simulink model "car_control"  (R2022b)
settings: Solver=VariableStepAuto  StartTime=0.0  StopTime=30  RelTol=1e-3
undefined symbols (not defined in the file): m, r
settings Model: Creator=The MathWorks, Inc.  LastModifiedBy=wzy19
settings SolverCC: AlgebraicLoopSolver=TrustRegion
settings DataIOCC: ReturnWorkspaceOutputs=off
settings DebuggingCC: BusObjectLabelMismatch=none  RootOutportRequireBusObject=none  PregeneratedLibrarySubsystemCodeDiagnostic=none  SFMachineParentedDataDiag=warning  ArithmeticOperatorsInVariantConditions=warning
settings ModelReferenceCC: EnableRefExpFcnMdlSchedulingChecks=on
settings SFSimCC: SimUseLocalCustomCode=off
settings RTWCC: RTWUseLocalCustomCode=off

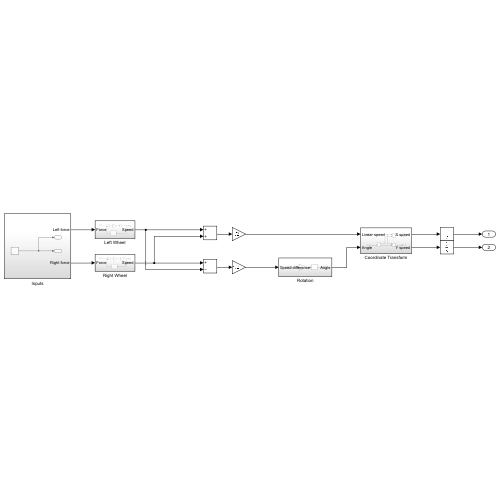
[thumbnail: Simulink's stored preview of the top-level diagram]
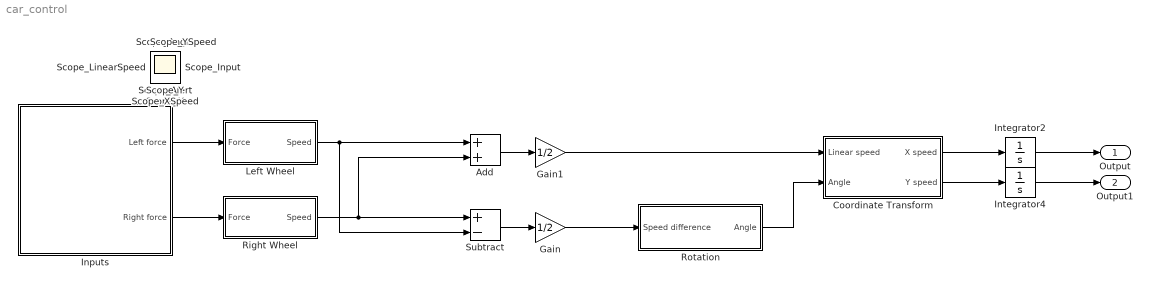
== system car_control ==
  Add : Sum
  Coordinate Transform : Subsystem
  Gain : Gain  Gain=1/2
  Gain1 : Gain  Gain=1/2
  Inputs : Subsystem
  Integrator2 : Integrator
  Integrator4 : Integrator
  Left Wheel : Subsystem
  Right Wheel : Subsystem
  Rotation : Subsystem
  Subtract : Sum  Inputs=+-
  Output : Outport
  Output1 : Outport  Port=2
  Scope_Alert : Scope
  Scope_Angle : Scope
  Scope_Input : Scope
  Scope_LinearSpeed : Scope
  Scope_X : Scope
  Scope_XSpeed : Scope
  Scope_Y : Scope
  Scope_YSpeed : Scope
  wires:
  Coordinate Transform/1(X speed) -> Integrator2/1
  Coordinate Transform/2(Y speed) -> Integrator4/1
  Left Wheel/1(Speed) -> Subtract/2, Add/1
  Right Wheel/1(Speed) -> Add/2, Subtract/1
  Subtract/1 -> Gain/1
  Gain/1 -> Rotation/1(Speed difference)
  Add/1 -> Gain1/1
  Gain1/1 -> Coordinate Transform/1(Linear speed)
  Rotation/1(Angle) -> Coordinate Transform/2(Angle)
  Inputs/1(Left force) -> Left Wheel/1(Force)
  Inputs/2(Right force) -> Right Wheel/1(Force)
  Integrator2/1 -> Output/1
  Integrator4/1 -> Output1/1

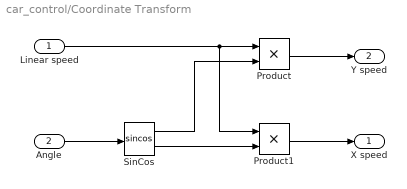
== system car_control/Coordinate Transform ==
  Linear speed : Inport
  Angle : Inport  Port=2
  Product : Product
  Product1 : Product
  SinCos : Trigonometry  Operator=sincos
  X speed : Outport  VectorParamsAs1DForOutWhenUnconnected=off
  Y speed : Outport  Port=2  VectorParamsAs1DForOutWhenUnconnected=off
  wires:
  Angle/1 -> SinCos/1
  SinCos/2 -> Product1/2
  SinCos/1 -> Product/2
  Linear speed/1 -> Product/1, Product1/1
  Product/1 -> Y speed/1
  Product1/1 -> X speed/1

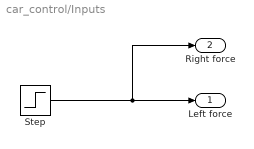
== system car_control/Inputs ==
  Step : Step  SampleTime=0
  Left force : Outport  VectorParamsAs1DForOutWhenUnconnected=off
  Right force : Outport  Port=2  VectorParamsAs1DForOutWhenUnconnected=off
  wires:
  Step/1 -> Right force/1, Left force/1

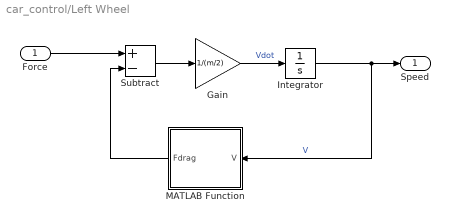
== system car_control/Left Wheel ==
  Force : Inport
  Gain : Gain  Gain=1/(m/2)
  Integrator : Integrator
  MATLAB Function : MATLAB Function  TreatAsAtomicUnit=on
  Subtract : Sum  Inputs=+-
  Speed : Outport  VectorParamsAs1DForOutWhenUnconnected=off
  wires:
  MATLAB Function/1(Fdrag) -> Subtract/2
  Subtract/1 -> Gain/1
  Gain/1 -> Integrator/1  "Vdot"
  Integrator/1 -> MATLAB Function/1(V), Speed/1  "V"
  Force/1 -> Subtract/1

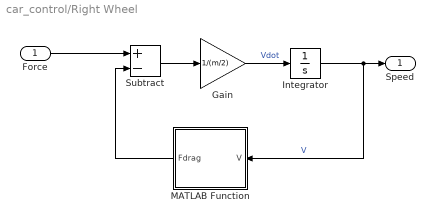
== system car_control/Right Wheel ==
  Force : Inport
  Gain : Gain  Gain=1/(m/2)
  Integrator : Integrator
  MATLAB Function : MATLAB Function  TreatAsAtomicUnit=on
  Subtract : Sum  Inputs=+-
  Speed : Outport  VectorParamsAs1DForOutWhenUnconnected=off
  wires:
  Integrator/1 -> MATLAB Function/1(V), Speed/1  "V"
  Subtract/1 -> Gain/1
  MATLAB Function/1(Fdrag) -> Subtract/2
  Gain/1 -> Integrator/1  "Vdot"
  Force/1 -> Subtract/1

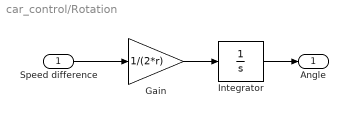
== system car_control/Rotation ==
  Speed difference : Inport
  Gain : Gain  Gain=1/(2*r)
  Integrator : Integrator
  Angle : Outport  VectorParamsAs1DForOutWhenUnconnected=off
  wires:
  Integrator/1 -> Angle/1
  Speed difference/1 -> Gain/1
  Gain/1 -> Integrator/1

== matlab function car_control/Right Wheel/MATLAB Function ==
  data: V input; Fdrag output; k_drag parameter
function Fdrag = get_fdrag(V,k_drag)

Fdrag = k_drag*V*abs(V);

== matlab function car_control/Left Wheel/MATLAB Function ==
  data: V input; Fdrag output; k_drag parameter
function Fdrag = get_fdrag(V,k_drag)

Fdrag = k_drag*V*abs(V);
